simulink model "Tracking"  (Simulink 8.9)
settings: Solver=VariableStepAuto  StartTime=0.0  StopTime=1  RelTol=1e-3
undefined symbols (not defined in the file): magnitude
libraries: commfilt2 x24, simulink x20, dspmtrx3 x12, dspswit3 x8
(part 1 of 2)
settings Model: SuppressorTable="22 serialization::archive 11 0 6 0 0 16 64 0 0 0 0 6 0 0 1 0 79 Tracking Loop/Tracking Loops/Tracking Loop2/PRN Generator /Counter Free-Running 0 6 0 0 2 8 0 0 0 0 6 40 SimulinkFixedPoint:util:Overflowoccurred 0 0 0 6 0  0  0 0 0 0 8 20160523 0 0 0 10 57 55 0 1 41 Simulink:DataType:WarningOverFlowDetected 0 0 0  0  8 20160523 0 10 57 55 0 1 1 0 79 Tracking Loop/Tracking Loops/Tracking Loop4/PRN Generator /Counter Free-Running 2 8 0 40 SimulinkFixedPoint:util:Overflowoccurred 0 0 0  0  8 20160523 0 10 57 55 0 1 41 Simulink:DataType:WarningOverFlowDetected 0 0 0  0  8 20160523 0 10 57 55 0 1 1 0 84 Tracking/Tracking Loop/Tracking Loops/Tracking Loop1/Oscillator/Counter Free-Running 2 8 0 40 SimulinkFixedPoint:util:Overflowoccurred 0 0 0  0  8 20160523 0 10 57 55 0 1 41 Simulink:DataType:WarningOverFlowDetected 0 0 0  0  8 20160523 0 10 57 55 0 1 1 0 75 Tracking Loop/Tracking Loops/Tracking Loop1/Oscillator/Counter Free-Running 2 8 0 40 SimulinkFixedPoint:util:Overflowoccurred 0 0 0  0  8 20160523 0 10 57 55 0 1 41 Simulink:DataType:WarningOverFlowDetected 0 0 0  0  8 20160523 0 10 57 55 0 1 1 0 88 Tracking/Tracking Loop/Tracking Loops/Tracking Loop1/PRN Generator /Counter Free-Running 2 8 0 40 SimulinkFixedPoint:util:Overflowoccurred 0 0 0  0  8 20160523 0 10 57 55 0 1 41 Simulink:DataType:WarningOverFlowDetected 0 0 0  0  8 20160523 0 10 57 55 0 1 1 0 75 Tracking Loop/Tracking Loops/Tracking Loop4/Oscillator/Counter Free-Running 2 8 0 40 SimulinkFixedPoint:util:Overflowoccurred 0 0 0  0  8 20160523 0 10 57 55 0 1 41 Simulink:DataType:WarningOverFlowDetected 0 0 0  0  8 20160523 0 10 57 55 0 1 1 0 79 Tracking Loop/Tracking Loops/Tracking Loop3/PRN Generator /Counter Free-Running 2 8 0 40 SimulinkFixedPoint:util:Overflowoccurred 0 0 0  0  8 20160523 0 10 57 55 0 1 41 Simulink:DataType:WarningOverFlowDetected 0 0 0  0  8 20160523 0 10 57 55 0 1 1 0 75 Tracking Loop/Tracking Loops/Tracking Loop3/Oscillator/Counter Free-Running 2 8 0 40 SimulinkFixedPoint:util:Overflowoccurred 0 0 0  0  8 20160523 0 10 57 55 0 1 41 Simulink:DataType:WarningOverFlowDetected 0 0 0  0  8 20160523 0 10 57 55 0 1 1 0 75 Tracking Loop/Tracking Loops/Tracking Loop2/Oscillator/Counter Free-Running 2 8 0 40 SimulinkFixedPoint:util:Overflowoccurred 0 0 0  0  8 20160523 0 10 57 55 0 1 41 Simulink:DataType:WarningOverFlowDetected 0 0 0  0  8 20160523 0 10 57 55 0 1 1 0 79 Tracking Loop/Tracking Loops/Tracking Loop1/PRN Generator /Counter Free-Running 2 8 0 40 SimulinkFixedPoint:util:Overflowoccurred 0 0 0  0  8 20160523 0 10 57 55 0 1 41 Simulink:DataType:WarningOverFlowDetected 0 0 0  0  8 20160523 0 10 57 55 0 1 1 0 84 Tracking/Tracking Loop/Tracking Loops/Tracking Loop2/Oscillator/Counter Free-Running 2 8 0 40 SimulinkFixedPoint:util:Overflowoccurred 0 0 0  0  8 20160523 0 10 57 55 0 1 41 Simulink:DataType:WarningOverFlowDetected 0 0 0  0  8 20160523 0 10 57 55 0 1 1 0 88 Tracking/Tracking Loop/Tracking Loops/Tracking Loop2/PRN Generator /Counter Free-Running 2 8 0 40 SimulinkFixedPoint:util:Overflowoccurred 0 0 0  0  8 20160523 0 10 57 55 0 1 41 Simulink:DataType:WarningOverFlowDetected 0 0 0  0  8 20160523 0 10 57 55 0 1 1 0 84 Tracking/Tracking Loop/Tracking Loops/Tracking Loop3/Oscillator/Counter Free-Running 2 8 0 40 SimulinkFixedPoint:util:Overflowoccurred 0 0 0  0  8 20160523 0 10 57 55 0 1 41 Simulink:DataType:WarningOverFlowDetected 0 0 0  0  8 20160523 0 10 57 55 0 1 1 0 88 Tracking/Tracking Loop/Tracking Loops/Tracking Loop3/PRN Generator /Counter Free-Running 2 8 0 40 SimulinkFixedPoint:util:Overflowoccurred 0 0 0  0  8 20160523 0 10 57 55 0 1 41 Simulink:DataType:WarningOverFlowDetected 0 0 0  0  8 20160523 0 10 57 55 0 1 1 0 84 Tracking/Tracking Loop/Tracking Loops/Tracking Loop4/Oscillator/Counter Free-Running 2 8 0 40 SimulinkFixedPoint:util:Overflowoccurred 0 0 0  0  8 20160523 0 10 57 55 0 1 41 Simulink:DataType:WarningOverFlowDetected 0 0 0  0  8 20160523 0 10 57 55 0 1 1 0 88 Tracking/Tracking Loop/Tracking Loops/Tracking Loop4/PRN Generator /Counter Free-Running 2 8 0 40 SimulinkFixedPoint:util:Overflowoccurred 0 0 0  0  8 20160523 0 10 57 55 0 1 41 Simulink:DataType:WarningOverFlowDetected 0 0 0  0  8 20160523 0 10 57 55 0 1"  Creator=Alam  LastModifiedBy=Alam
settings DataIOCC: LimitDataPoints=off  SaveFormat=Dataset  SignalLoggingSaveFormat=Dataset
settings OptimizationCC: LifeSpan=auto
settings DebuggingCC: UnderspecifiedInitializationDetection=Simplified  MergeDetectMultiDrivingBlocksExec=error  FcnCallInpInsideContextMsg=error  StateNameClashWarn=none  SFUnexpectedBacktrackingDiag=error  SFNoUnconditionalDefaultTransitionDiag=error  SFExecutionAtInitializationDiag=warning
settings HardwareCC: ProdBitPerPointer=64  ProdBitPerSizeT=64  ProdBitPerPtrDiffT=64  ProdLargestAtomicFloat=Float  ProdIntDivRoundTo=Zero  ProdEndianess=LittleEndian  ProdWordSize=64  ProdHWDeviceType=Intel->x86-64 (Windows64)
settings ModelReferenceCC: PropagateSignalLabelsOutOfModel=on
settings GRTTargetCC: TargetLangStandard=C99 (ISO)  GeneratePreprocessorConditionals=Use local settings  CombineOutputUpdateFcns=on  GRTInterface=off
settings ConfigComp: CovMetricSettings=dwe  CovHtmlReporting=off  CovSaveCumulativeToWorkspaceVar=off  CovSaveSingleToWorkspaceVar=off  CovExternalEMLEnable=on

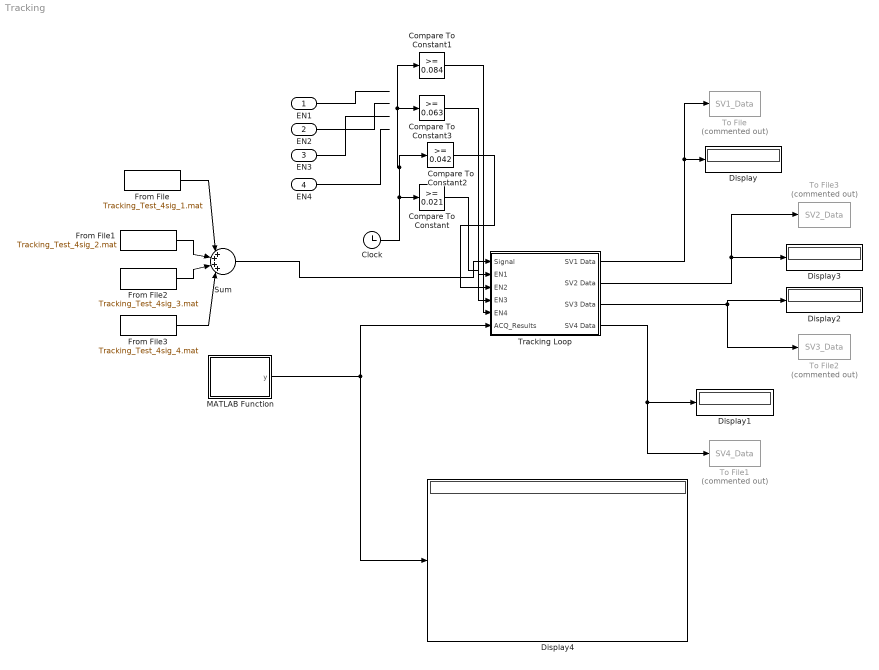
== system Tracking ==
  EN1 : Inport
  EN2 : Inport  Port=2
  EN3 : Inport  Port=3
  EN4 : Inport  Port=4
  Clock : Clock
  Compare To Constant : simulink/Logic and Bit Operations/Compare To Constant  relop=>=  const=0.021  OutDataTypeStr=boolean
  Compare To Constant1 : simulink/Logic and Bit Operations/Compare To Constant  relop=>=  const=0.084  OutDataTypeStr=boolean
  Compare To Constant2 : simulink/Logic and Bit Operations/Compare To Constant  relop=>=  const=0.042  OutDataTypeStr=boolean
  Compare To Constant3 : simulink/Logic and Bit Operations/Compare To Constant  relop=>=  const=0.063  OutDataTypeStr=boolean
  Display{,1..4} (5 alike) : Display
  From File : FromFile  FileName=Tracking_Test_4sig_1.mat  SampleTime=0
  From File1 : FromFile  FileName=Tracking_Test_4sig_2.mat  SampleTime=0
  From File2 : FromFile  FileName=Tracking_Test_4sig_3.mat  SampleTime=0
  From File3 : FromFile  FileName=Tracking_Test_4sig_4.mat  SampleTime=0
  MATLAB Function : MATLAB Function
  Sum : Sum  Inputs=|++++|
  To File : ToFile  Commented=on  Filename=SV1_Data  MatrixName=SV1  SampleTime=0.01
  To File1 : ToFile  Commented=on  Filename=SV4_Data  MatrixName=SV4  SampleTime=0.01
  To File2 : ToFile  Commented=on  Filename=SV3_Data  MatrixName=SV3  SampleTime=0.01
  To File3 : ToFile  Commented=on  Filename=SV2_Data  MatrixName=SV2  SampleTime=0.01
  Tracking Loop : Subsystem  TreatAsAtomicUnit=on
  wires:
  Tracking Loop/3(SV3 Data) -> Display2/1, To File2/1
  Tracking Loop/4(SV4 Data) -> To File1/1, Display1/1
  Tracking Loop/2(SV2 Data) -> Display3/1, To File3/1
  Tracking Loop/1(SV1 Data) -> Display/1, To File/1
  Compare To Constant2/1 -> Tracking Loop/3(EN2)
  Compare To Constant/1 -> Tracking Loop/2(EN1)
  Clock/1 -> Compare To Constant1/1, Compare To Constant3/1, Compare To Constant2/1, Compare To Constant/1
  Compare To Constant3/1 -> Tracking Loop/4(EN3)
  Compare To Constant1/1 -> Tracking Loop/5(EN4)
  Sum/1 -> Tracking Loop/1(Signal)
  From File2/1 -> Sum/3
  From File/1 -> Sum/1
  From File1/1 -> Sum/2
  From File3/1 -> Sum/4
  EN3/1 -> ?
  EN4/1 -> ?
  EN2/1 -> ?
  EN1/1 -> ?
  MATLAB Function/1(y) -> Tracking Loop/6(ACQ_Results), Display4/1

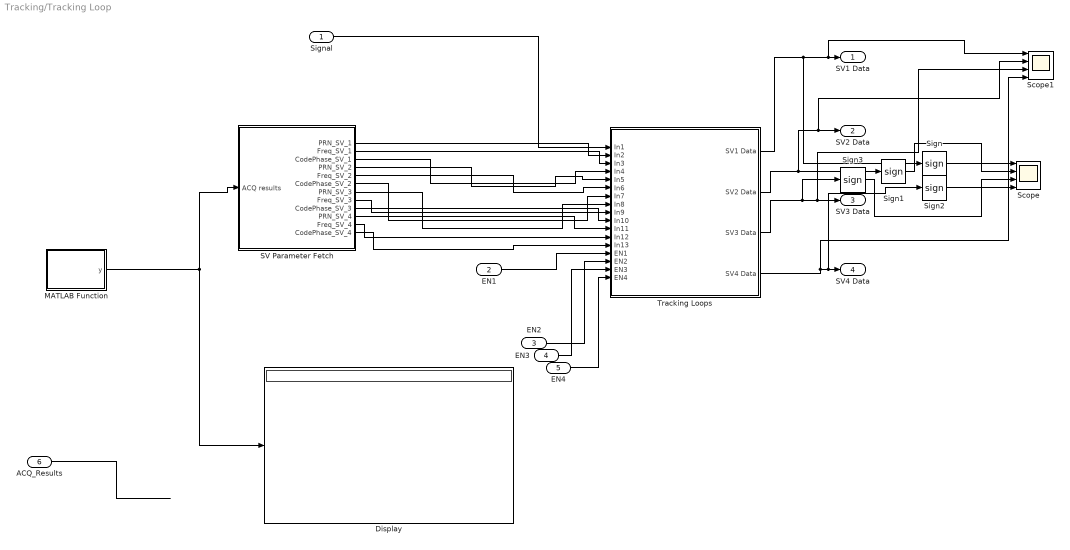
== system Tracking/Tracking Loop ==
  Signal : Inport
  EN1 : Inport  Port=2
  EN2 : Inport  Port=3
  EN3 : Inport  Port=4
  EN4 : Inport  Port=5
  ACQ_Results : Inport  Port=6
  Display : Display
  MATLAB Function : MATLAB Function  TreatAsAtomicUnit=on
  SV Parameter Fetch : Subsystem
  Scope : Scope  NumInputPorts=4
  Scope1 : Scope  NumInputPorts=4
  Sign{,1..3} (4 alike) : Signum
  Tracking Loops : Subsystem
  SV1 Data : Outport
  SV2 Data : Outport  Port=2
  SV3 Data : Outport  Port=3
  SV4 Data : Outport  Port=4
  wires:
  Signal/1 -> Tracking Loops/1(In1)
  Tracking Loops/1(SV1 Data) -> Sign/1, Scope1/1, SV1 Data/1
  Tracking Loops/2(SV2 Data) -> Scope1/2, SV2 Data/1, Sign1/1
  Tracking Loops/3(SV3 Data) -> Sign3/1, Scope1/3, SV3 Data/1
  Tracking Loops/4(SV4 Data) -> Scope1/4, Sign2/1, SV4 Data/1
  Sign/1 -> Scope/1
  Sign1/1 -> Scope/2
  Sign2/1 -> Scope/4
  Sign3/1 -> Scope/3
  SV Parameter Fetch/12(CodePhase_SV_4) -> Tracking Loops/13(In13)
  SV Parameter Fetch/11(Freq_SV_4) -> Tracking Loops/12(In12)
  SV Parameter Fetch/10(PRN_SV_4) -> Tracking Loops/11(In11)
  SV Parameter Fetch/9(CodePhase_SV_3) -> Tracking Loops/10(In10)
  SV Parameter Fetch/8(Freq_SV_3) -> Tracking Loops/9(In9)
  SV Parameter Fetch/7(PRN_SV_3) -> Tracking Loops/8(In8)
  SV Parameter Fetch/6(CodePhase_SV_2) -> Tracking Loops/7(In7)
  SV Parameter Fetch/5(Freq_SV_2) -> Tracking Loops/6(In6)
  SV Parameter Fetch/4(PRN_SV_2) -> Tracking Loops/5(In5)
  SV Parameter Fetch/3(CodePhase_SV_1) -> Tracking Loops/4(In4)
  SV Parameter Fetch/2(Freq_SV_1) -> Tracking Loops/3(In3)
  SV Parameter Fetch/1(PRN_SV_1) -> Tracking Loops/2(In2)
  MATLAB Function/1(y) -> SV Parameter Fetch/1(ACQ results), Display/1
  EN1/1 -> Tracking Loops/14(EN1)
  EN2/1 -> Tracking Loops/15(EN2)
  EN3/1 -> Tracking Loops/16(EN3)
  EN4/1 -> Tracking Loops/17(EN4)
  ACQ_Results/1 -> ?

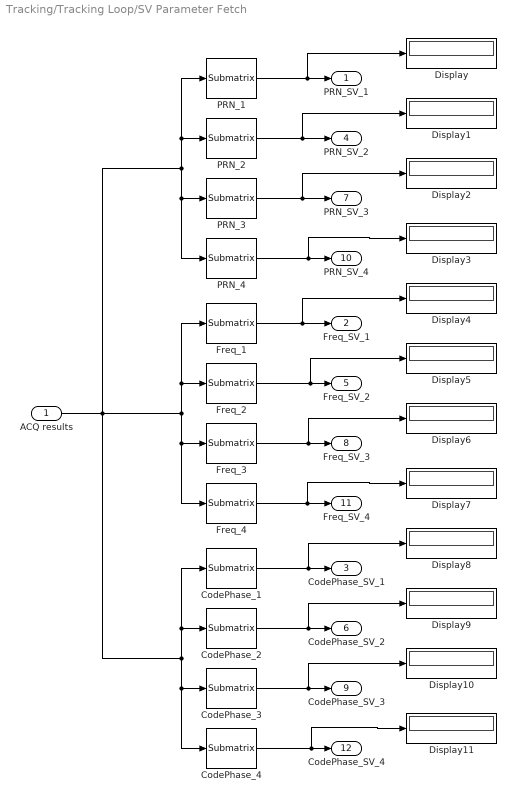
== system Tracking/Tracking Loop/SV Parameter Fetch ==
  ACQ results : Inport
  CodePhase_1 : dspmtrx3/Submatrix  RowSpan=One row  RowStartMode=Index  RowStartIndex=1  RowEndMode=Last  RowEndIndex=1  ColSpan=One column  ColStartMode=Index  ColStartIndex=4  ColEndMode=Last  ColEndIndex=1
  CodePhase_2 : dspmtrx3/Submatrix  RowSpan=One row  RowStartMode=Index  RowStartIndex=2  RowEndMode=Last  RowEndIndex=1  ColSpan=One column  ColStartMode=Index  ColStartIndex=4  ColEndMode=Last  ColEndIndex=1
  CodePhase_3 : dspmtrx3/Submatrix  RowSpan=One row  RowStartMode=Index  RowStartIndex=3  RowEndMode=Last  RowEndIndex=1  ColSpan=One column  ColStartMode=Index  ColStartIndex=4  ColEndMode=Last  ColEndIndex=1
  CodePhase_4 : dspmtrx3/Submatrix  RowSpan=One row  RowStartMode=Index  RowStartIndex=4  RowEndMode=Last  RowEndIndex=1  ColSpan=One column  ColStartMode=Index  ColStartIndex=4  ColEndMode=Last  ColEndIndex=1
  Display{,1..11} (12 alike) : Display
  Freq_1 : dspmtrx3/Submatrix  RowSpan=One row  RowStartMode=Index  RowStartIndex=1  RowEndMode=Last  RowEndIndex=1  ColSpan=One column  ColStartMode=Index  ColStartIndex=3  ColEndMode=Last  ColEndIndex=1
  Freq_2 : dspmtrx3/Submatrix  RowSpan=One row  RowStartMode=Index  RowStartIndex=2  RowEndMode=Last  RowEndIndex=1  ColSpan=One column  ColStartMode=Index  ColStartIndex=3  ColEndMode=Last  ColEndIndex=1
  Freq_3 : dspmtrx3/Submatrix  RowSpan=One row  RowStartMode=Index  RowStartIndex=3  RowEndMode=Last  RowEndIndex=1  ColSpan=One column  ColStartMode=Index  ColStartIndex=3  ColEndMode=Last  ColEndIndex=1
  Freq_4 : dspmtrx3/Submatrix  RowSpan=One row  RowStartMode=Index  RowStartIndex=4  RowEndMode=Last  RowEndIndex=1  ColSpan=One column  ColStartMode=Index  ColStartIndex=3  ColEndMode=Last  ColEndIndex=1
  PRN_1 : dspmtrx3/Submatrix  RowSpan=One row  RowStartMode=Index  RowStartIndex=1  RowEndMode=Last  RowEndIndex=1  ColSpan=One column  ColStartMode=Index  ColStartIndex=2  ColEndMode=Last  ColEndIndex=1
  PRN_2 : dspmtrx3/Submatrix  RowSpan=One row  RowStartMode=Index  RowStartIndex=2  RowEndMode=Last  RowEndIndex=1  ColSpan=One column  ColStartMode=Index  ColStartIndex=2  ColEndMode=Last  ColEndIndex=1
  PRN_3 : dspmtrx3/Submatrix  RowSpan=One row  RowStartMode=Index  RowStartIndex=3  RowEndMode=Last  RowEndIndex=1  ColSpan=One column  ColStartMode=Index  ColStartIndex=2  ColEndMode=Last  ColEndIndex=1
  PRN_4 : dspmtrx3/Submatrix  RowSpan=One row  RowStartMode=Index  RowStartIndex=4  RowEndMode=Last  RowEndIndex=1  ColSpan=One column  ColStartMode=Index  ColStartIndex=2  ColEndMode=Last  ColEndIndex=1
  PRN_SV_1 : Outport
  Freq_SV_1 : Outport  Port=2
  CodePhase_SV_1 : Outport  Port=3
  PRN_SV_2 : Outport  Port=4
  Freq_SV_2 : Outport  Port=5
  CodePhase_SV_2 : Outport  Port=6
  PRN_SV_3 : Outport  Port=7
  Freq_SV_3 : Outport  Port=8
  CodePhase_SV_3 : Outport  Port=9
  PRN_SV_4 : Outport  Port=10
  Freq_SV_4 : Outport  Port=11
  CodePhase_SV_4 : Outport  Port=12
  wires:
  ACQ results/1 -> CodePhase_4/1, CodePhase_3/1, CodePhase_2/1, CodePhase_1/1, Freq_4/1, Freq_3/1, Freq_2/1, Freq_1/1, PRN_4/1, PRN_3/1, PRN_2/1, PRN_1/1
  PRN_1/1 -> Display/1, PRN_SV_1/1
  PRN_2/1 -> Display1/1, PRN_SV_2/1
  PRN_3/1 -> Display2/1, PRN_SV_3/1
  PRN_4/1 -> Display3/1, PRN_SV_4/1
  Freq_1/1 -> Display4/1, Freq_SV_1/1
  Freq_2/1 -> Display5/1, Freq_SV_2/1
  Freq_3/1 -> Display6/1, Freq_SV_3/1
  Freq_4/1 -> Display7/1, Freq_SV_4/1
  CodePhase_1/1 -> Display8/1, CodePhase_SV_1/1
  CodePhase_2/1 -> Display9/1, CodePhase_SV_2/1
  CodePhase_3/1 -> Display10/1, CodePhase_SV_3/1
  CodePhase_4/1 -> Display11/1, CodePhase_SV_4/1

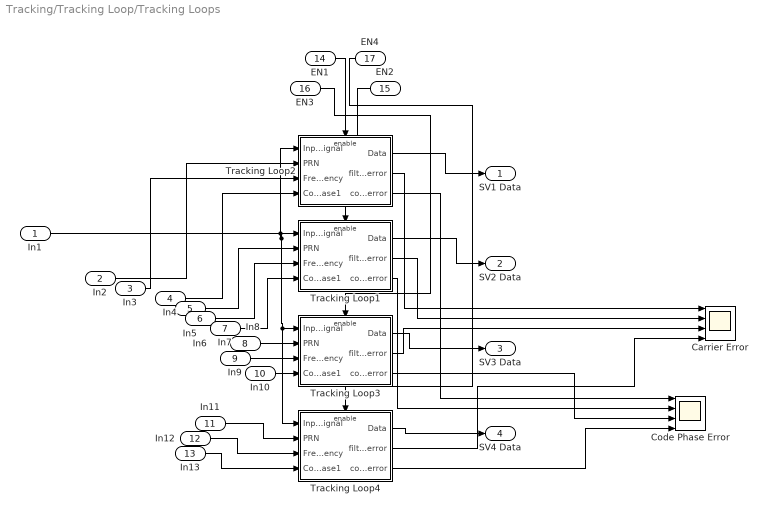
== system Tracking/Tracking Loop/Tracking Loops ==
  In1 : Inport
  In2 : Inport  Port=2
  In3 : Inport  Port=3
  In4 : Inport  Port=4
  In5 : Inport  Port=5
  In6 : Inport  Port=6
  In7 : Inport  Port=7
  In8 : Inport  Port=8
  In9 : Inport  Port=9
  In10 : Inport  Port=10
  In11 : Inport  Port=11
  In12 : Inport  Port=12
  In13 : Inport  Port=13
  EN1 : Inport  Port=14
  EN2 : Inport  Port=15
  EN3 : Inport  Port=16
  EN4 : Inport  Port=17
  Carrier Error : Scope  NumInputPorts=4
  Code Phase Error : Scope  NumInputPorts=4
  Tracking Loop1 : Subsystem  TreatAsAtomicUnit=on
      settings: PropExecContextOutsideSubsystem=on
  Tracking Loop2 : Subsystem  TreatAsAtomicUnit=on
  Tracking Loop3 : Subsystem  TreatAsAtomicUnit=on
      settings: PropExecContextOutsideSubsystem=on
  Tracking Loop4 : Subsystem  TreatAsAtomicUnit=on
      settings: PropExecContextOutsideSubsystem=on
  SV1 Data : Outport
  SV2 Data : Outport  Port=2
  SV3 Data : Outport  Port=3
  SV4 Data : Outport  Port=4
  wires:
  In1/1 -> Tracking Loop2/1(Input Signal), Tracking Loop1/1(Input Signal), Tracking Loop4/1(Input Signal), Tracking Loop3/1(Input Signal)
  Tracking Loop2/1(Data) -> SV1 Data/1
  Tracking Loop4/1(Data) -> SV4 Data/1
  Tracking Loop3/1(Data) -> SV3 Data/1
  In12/1 -> Tracking Loop4/3(Frequency)
  In3/1 -> Tracking Loop2/3(Frequency)
  In4/1 -> Tracking Loop2/4(Code Phase1)
  In6/1 -> Tracking Loop1/3(Frequency)
  In13/1 -> Tracking Loop4/4(Code Phase1)
  In9/1 -> Tracking Loop3/3(Frequency)
  In8/1 -> Tracking Loop3/2(PRN)
  In11/1 -> Tracking Loop4/2(PRN)
  In5/1 -> Tracking Loop1/2(PRN)
  In10/1 -> Tracking Loop3/4(Code Phase1)
  In2/1 -> Tracking Loop2/2(PRN)
  In7/1 -> Tracking Loop1/4(Code Phase1)
  Tracking Loop1/1(Data) -> SV2 Data/1
  Tracking Loop2/2(filter error) -> Carrier Error/1
  Tracking Loop1/2(filter error) -> Carrier Error/2
  Tracking Loop3/2(filter error) -> Carrier Error/3
  Tracking Loop4/2(filter error) -> Carrier Error/4
  Tracking Loop3/3(code_phase_error) -> Code Phase Error/3
  Tracking Loop4/3(code_phase_error) -> Code Phase Error/4
  Tracking Loop2/3(code_phase_error) -> Code Phase Error/1
  Tracking Loop1/3(code_phase_error) -> Code Phase Error/2
  EN1/1 -> Tracking Loop2/Enable
  EN2/1 -> Tracking Loop1/Enable
  EN3/1 -> Tracking Loop3/Enable
  EN4/1 -> Tracking Loop4/Enable

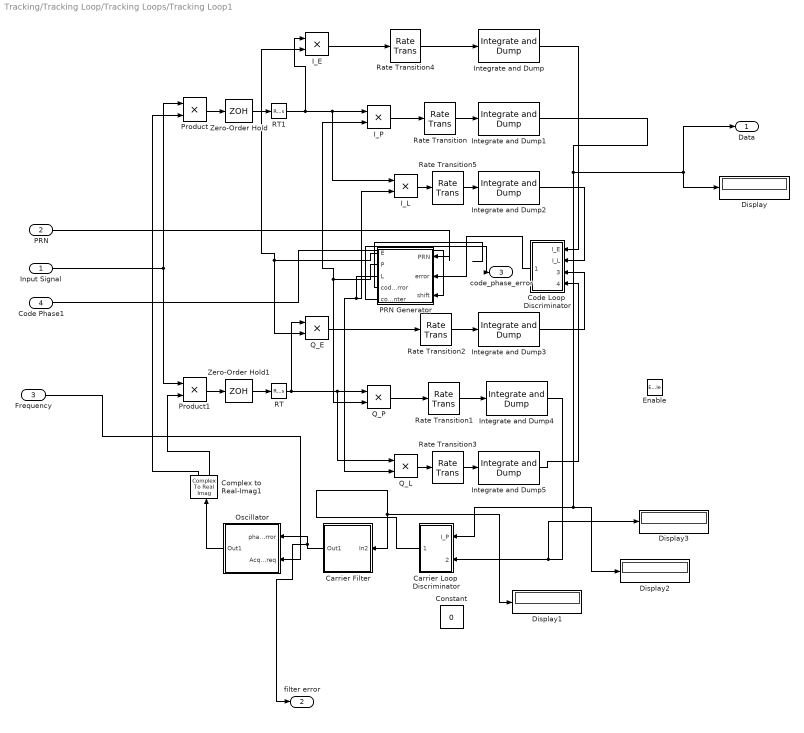
== system Tracking/Tracking Loop/Tracking Loops/Tracking Loop1 ==
  Input Signal : Inport
  PRN : Inport  Port=2
  Frequency : Inport  Port=3
  Code Phase1 : Inport  Port=4
  Enable : EnablePort
  Carrier Filter : Subsystem
  "Carrier Loop  Discriminator " : Subsystem
  Code Loop  Discriminator : Subsystem
  Complex to Real-Imag1 : ComplexToRealImag
  Constant : Constant  Value=0  SampleTime=0.001
  Display{,1..3} (4 alike) : Display
  I_E : Product
  I_L : Product
  "I_P " : Product
  Integrate and Dump{,1..5} (6 alike) : commfilt2/Integrate and Dump  obssamples=32768  offsetsamples=0  nodump=off  roundingMode=Floor  overflowMode=off  outputDataTypeStr=Inherit: Same as accumulator  outputLastDataTypeStr=Inherit: Same as accumulator
      settings: SourceProductName=Communications System Toolbox
  Oscillator : Subsystem
  "PRN Generator " : Subsystem
  Product : Product
  Product1 : Product
  Q_E : Product
  Q_L : Product
  Q_P : Product
  RT : RateTransition
  RT1 : RateTransition
  Rate Transition{,1..5} (6 alike) : RateTransition  OutPortSampleTime=3.0517578125e-8
  Zero-Order Hold : ZeroOrderHold  SampleTime=3.0517578125e-8
  Zero-Order Hold1 : ZeroOrderHold  SampleTime=3.0517578125e-8
  Data : Outport
  filter error : Outport  Port=2
  code_phase_error : Outport  Port=3
  wires:
  I_L/1 -> Rate Transition5/1
  "PRN Generator "/3(L) -> Q_L/2, I_L/2
  Q_E/1 -> Rate Transition2/1
  Q_L/1 -> Rate Transition3/1
  "PRN Generator "/2(P) -> "I_P "/2, Q_P/2
  Q_P/1 -> Rate Transition1/1
  "I_P "/1 -> Rate Transition/1
  "Carrier Loop  Discriminator "/1(theta) -> Carrier Filter/1(In2), Display1/1
  Rate Transition/1 -> Integrate and Dump1/1
  Rate Transition4/1 -> Integrate and Dump/1
  RT/1 -> Q_L/1, Q_P/1, Q_E/1
  Code Phase1/1 -> "PRN Generator "/3(shift)
  Product/1 -> Zero-Order Hold/1
  PRN/1 -> "PRN Generator "/1(PRN)
  Complex to Real-Imag1/2 -> Product1/2
  Input Signal/1 -> Product1/1, Product/1
  Complex to Real-Imag1/1 -> Product/2
  I_E/1 -> Rate Transition4/1
  Integrate and Dump/1 -> Code Loop  Discriminator/1(I_E)
  Integrate and Dump5/1 -> Code Loop  Discriminator/4(Q_L)
  Integrate and Dump3/1 -> Code Loop  Discriminator/3(Q_E)
  "PRN Generator "/1(E) -> I_E/2, Q_E/2
  Integrate and Dump2/1 -> Code Loop  Discriminator/2(I_L)
  Rate Transition1/1 -> Integrate and Dump4/1
  Rate Transition3/1 -> Integrate and Dump5/1
  Rate Transition2/1 -> Integrate and Dump3/1
  Rate Transition5/1 -> Integrate and Dump2/1
  Frequency/1 -> Oscillator/2(Acq Freq)
  Product1/1 -> Zero-Order Hold1/1
  Zero-Order Hold/1 -> RT1/1
  RT1/1 -> I_E/1, I_L/1, "I_P "/1
  Zero-Order Hold1/1 -> RT/1
  Oscillator/1(Out1) -> Complex to Real-Imag1/1
  Carrier Filter/1(Out1) -> filter error/1, Oscillator/1(phase error)
  Integrate and Dump4/1 -> "Carrier Loop  Discriminator "/2(Q_P), Display3/1
  Integrate and Dump1/1 -> Display/1, Data/1, "Carrier Loop  Discriminator "/1(I_P), Display2/1
  "PRN Generator "/4(code_phase_error) -> ?
  "PRN Generator "/5(code_phase_counter) -> code_phase_error/1
  Code Loop  Discriminator/1(error) -> "PRN Generator "/2(error)

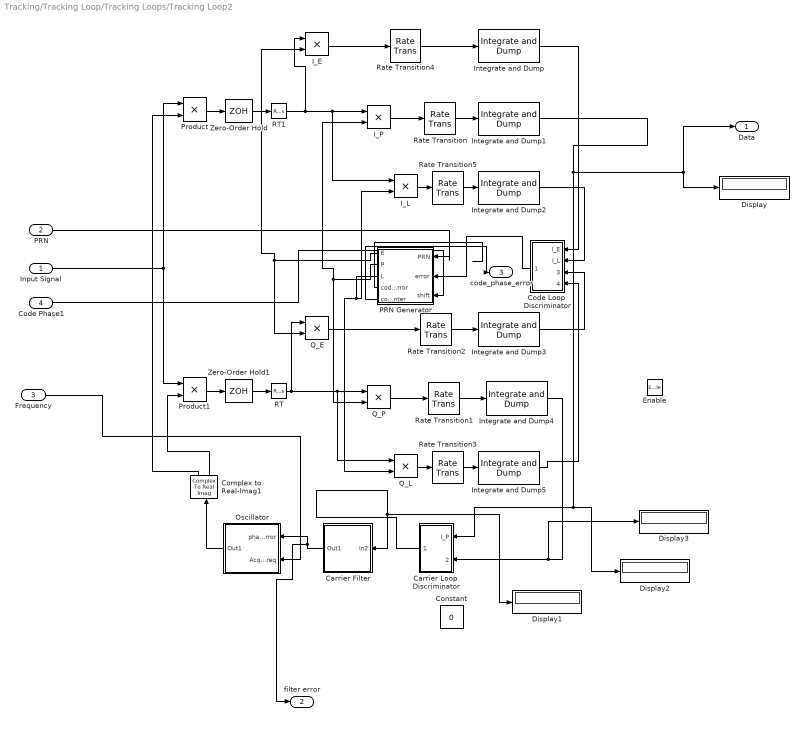
== system Tracking/Tracking Loop/Tracking Loops/Tracking Loop2 ==
  Input Signal : Inport
  PRN : Inport  Port=2
  Frequency : Inport  Port=3
  Code Phase1 : Inport  Port=4
  Enable : EnablePort
  Carrier Filter : Subsystem
      settings: MinAlgLoopOccurrences=on
  "Carrier Loop  Discriminator " : Subsystem
  Code Loop  Discriminator : Subsystem
      settings: MinAlgLoopOccurrences=on
  Complex to Real-Imag1 : ComplexToRealImag
  Constant : Constant  Value=0  SampleTime=0.001
  Display{,1..3} (4 alike) : Display
  I_E : Product
  I_L : Product
  "I_P " : Product
  Integrate and Dump{,1..5} (6 alike) : commfilt2/Integrate and Dump  obssamples=32768  offsetsamples=0  nodump=off  roundingMode=Floor  overflowMode=off  outputDataTypeStr=Inherit: Same as accumulator  outputLastDataTypeStr=Inherit: Same as accumulator
      settings: SourceProductName=Communications System Toolbox
  Oscillator : Subsystem
  "PRN Generator " : Subsystem
      settings: MinAlgLoopOccurrences=on
  Product : Product
  Product1 : Product
  Q_E : Product
  Q_L : Product
  Q_P : Product
  RT : RateTransition
  RT1 : RateTransition
  Rate Transition{,1..5} (6 alike) : RateTransition  OutPortSampleTime=3.0517578125e-8
  Zero-Order Hold : ZeroOrderHold  SampleTime=3.0517578125e-8
  Zero-Order Hold1 : ZeroOrderHold  SampleTime=3.0517578125e-8
  Data : Outport
  filter error : Outport  Port=2
  code_phase_error : Outport  Port=3
  wires:
  I_L/1 -> Rate Transition5/1
  "PRN Generator "/3(L) -> Q_L/2, I_L/2
  Q_E/1 -> Rate Transition2/1
  Q_L/1 -> Rate Transition3/1
  "PRN Generator "/2(P) -> "I_P "/2, Q_P/2
  Q_P/1 -> Rate Transition1/1
  "I_P "/1 -> Rate Transition/1
  "Carrier Loop  Discriminator "/1(theta) -> Carrier Filter/1(In2), Display1/1
  Rate Transition/1 -> Integrate and Dump1/1
  Rate Transition4/1 -> Integrate and Dump/1
  RT/1 -> Q_L/1, Q_P/1, Q_E/1
  Code Phase1/1 -> "PRN Generator "/3(shift)
  Product/1 -> Zero-Order Hold/1
  PRN/1 -> "PRN Generator "/1(PRN)
  Complex to Real-Imag1/2 -> Product1/2
  Input Signal/1 -> Product1/1, Product/1
  Complex to Real-Imag1/1 -> Product/2
  I_E/1 -> Rate Transition4/1
  Integrate and Dump/1 -> Code Loop  Discriminator/1(I_E)
  Integrate and Dump5/1 -> Code Loop  Discriminator/4(Q_L)
  Integrate and Dump3/1 -> Code Loop  Discriminator/3(Q_E)
  "PRN Generator "/1(E) -> I_E/2, Q_E/2
  Integrate and Dump2/1 -> Code Loop  Discriminator/2(I_L)
  Rate Transition1/1 -> Integrate and Dump4/1
  Rate Transition3/1 -> Integrate and Dump5/1
  Rate Transition2/1 -> Integrate and Dump3/1
  Rate Transition5/1 -> Integrate and Dump2/1
  Frequency/1 -> Oscillator/2(Acq Freq)
  Product1/1 -> Zero-Order Hold1/1
  Zero-Order Hold/1 -> RT1/1
  RT1/1 -> I_E/1, I_L/1, "I_P "/1
  Zero-Order Hold1/1 -> RT/1
  Oscillator/1(Out1) -> Complex to Real-Imag1/1
  Carrier Filter/1(Out1) -> filter error/1, Oscillator/1(phase error)
  Integrate and Dump4/1 -> "Carrier Loop  Discriminator "/2(Q_P), Display3/1
  Integrate and Dump1/1 -> Display/1, Data/1, "Carrier Loop  Discriminator "/1(I_P), Display2/1
  "PRN Generator "/4(code_phase_error) -> ?
  "PRN Generator "/5(code_phase_counter) -> code_phase_error/1
  Code Loop  Discriminator/1(error) -> "PRN Generator "/2(error)

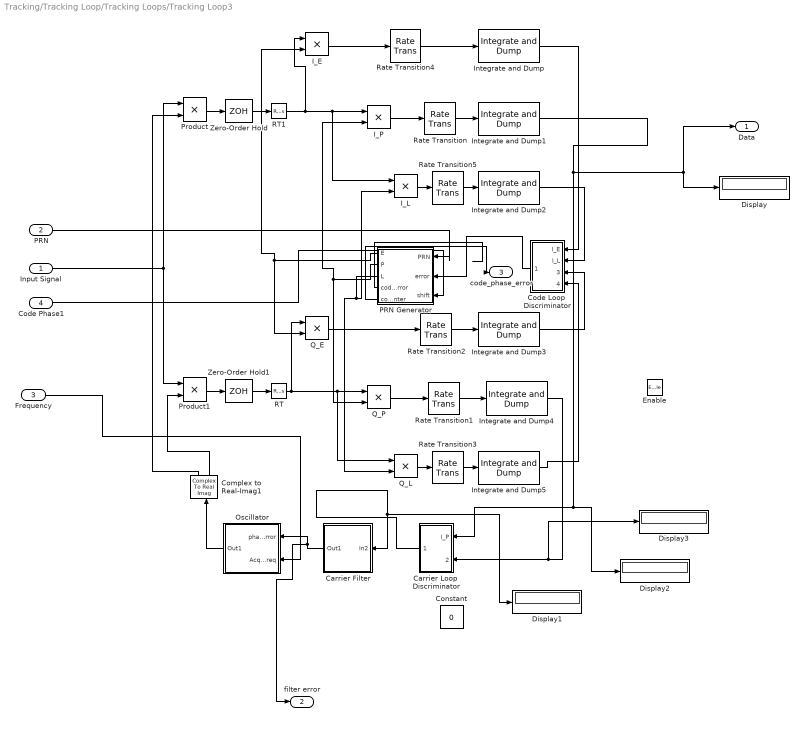
== system Tracking/Tracking Loop/Tracking Loops/Tracking Loop3 ==
  Input Signal : Inport
  PRN : Inport  Port=2
  Frequency : Inport  Port=3
  Code Phase1 : Inport  Port=4
  Enable : EnablePort
  Carrier Filter : Subsystem
  "Carrier Loop  Discriminator " : Subsystem
  Code Loop  Discriminator : Subsystem
  Complex to Real-Imag1 : ComplexToRealImag
  Constant : Constant  Value=0  SampleTime=0.001
  Display{,1..3} (4 alike) : Display
  I_E : Product
  I_L : Product
  "I_P " : Product
  Integrate and Dump{,1..5} (6 alike) : commfilt2/Integrate and Dump  obssamples=32768  offsetsamples=0  nodump=off  roundingMode=Floor  overflowMode=off  outputDataTypeStr=Inherit: Same as accumulator  outputLastDataTypeStr=Inherit: Same as accumulator
      settings: SourceProductName=Communications System Toolbox
  Oscillator : Subsystem
  "PRN Generator " : Subsystem
  Product : Product
  Product1 : Product
  Q_E : Product
  Q_L : Product
  Q_P : Product
  RT : RateTransition
  RT1 : RateTransition
  Rate Transition{,1..5} (6 alike) : RateTransition  OutPortSampleTime=3.0517578125e-8
  Zero-Order Hold : ZeroOrderHold  SampleTime=3.0517578125e-8
  Zero-Order Hold1 : ZeroOrderHold  SampleTime=3.0517578125e-8
  Data : Outport
  filter error : Outport  Port=2
  code_phase_error : Outport  Port=3
  wires:
  I_L/1 -> Rate Transition5/1
  "PRN Generator "/3(L) -> Q_L/2, I_L/2
  Q_E/1 -> Rate Transition2/1
  Q_L/1 -> Rate Transition3/1
  "PRN Generator "/2(P) -> "I_P "/2, Q_P/2
  Q_P/1 -> Rate Transition1/1
  "I_P "/1 -> Rate Transition/1
  "Carrier Loop  Discriminator "/1(theta) -> Carrier Filter/1(In2), Display1/1
  Rate Transition/1 -> Integrate and Dump1/1
  Rate Transition4/1 -> Integrate and Dump/1
  RT/1 -> Q_L/1, Q_P/1, Q_E/1
  Code Phase1/1 -> "PRN Generator "/3(shift)
  Product/1 -> Zero-Order Hold/1
  PRN/1 -> "PRN Generator "/1(PRN)
  Complex to Real-Imag1/2 -> Product1/2
  Input Signal/1 -> Product1/1, Product/1
  Complex to Real-Imag1/1 -> Product/2
  I_E/1 -> Rate Transition4/1
  Integrate and Dump/1 -> Code Loop  Discriminator/1(I_E)
  Integrate and Dump5/1 -> Code Loop  Discriminator/4(Q_L)
  Integrate and Dump3/1 -> Code Loop  Discriminator/3(Q_E)
  "PRN Generator "/1(E) -> I_E/2, Q_E/2
  Integrate and Dump2/1 -> Code Loop  Discriminator/2(I_L)
  Rate Transition1/1 -> Integrate and Dump4/1
  Rate Transition3/1 -> Integrate and Dump5/1
  Rate Transition2/1 -> Integrate and Dump3/1
  Rate Transition5/1 -> Integrate and Dump2/1
  Frequency/1 -> Oscillator/2(Acq Freq)
  Product1/1 -> Zero-Order Hold1/1
  Zero-Order Hold/1 -> RT1/1
  RT1/1 -> I_E/1, I_L/1, "I_P "/1
  Zero-Order Hold1/1 -> RT/1
  Oscillator/1(Out1) -> Complex to Real-Imag1/1
  Carrier Filter/1(Out1) -> filter error/1, Oscillator/1(phase error)
  Integrate and Dump4/1 -> "Carrier Loop  Discriminator "/2(Q_P), Display3/1
  Integrate and Dump1/1 -> Display/1, Data/1, "Carrier Loop  Discriminator "/1(I_P), Display2/1
  "PRN Generator "/4(code_phase_error) -> ?
  "PRN Generator "/5(code_phase_counter) -> code_phase_error/1
  Code Loop  Discriminator/1(error) -> "PRN Generator "/2(error)

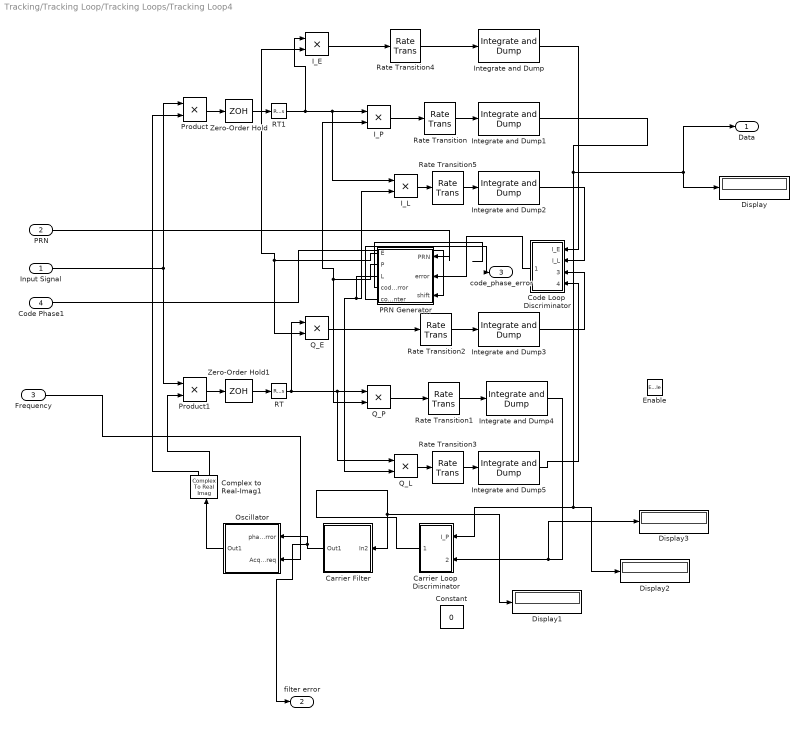
== system Tracking/Tracking Loop/Tracking Loops/Tracking Loop4 ==
  Input Signal : Inport
  PRN : Inport  Port=2
  Frequency : Inport  Port=3
  Code Phase1 : Inport  Port=4
  Enable : EnablePort
  Carrier Filter : Subsystem
  "Carrier Loop  Discriminator " : Subsystem
  Code Loop  Discriminator : Subsystem
  Complex to Real-Imag1 : ComplexToRealImag
  Constant : Constant  Value=0  SampleTime=0.001
  Display{,1..3} (4 alike) : Display
  I_E : Product
  I_L : Product
  "I_P " : Product
  Integrate and Dump{,1..5} (6 alike) : commfilt2/Integrate and Dump  obssamples=32768  offsetsamples=0  nodump=off  roundingMode=Floor  overflowMode=off  outputDataTypeStr=Inherit: Same as accumulator  outputLastDataTypeStr=Inherit: Same as accumulator
      settings: SourceProductName=Communications System Toolbox
  Oscillator : Subsystem
  "PRN Generator " : Subsystem
  Product : Product
  Product1 : Product
  Q_E : Product
  Q_L : Product
  Q_P : Product
  RT : RateTransition
  RT1 : RateTransition
  Rate Transition{,1..5} (6 alike) : RateTransition  OutPortSampleTime=3.0517578125e-8
  Zero-Order Hold : ZeroOrderHold  SampleTime=3.0517578125e-8
  Zero-Order Hold1 : ZeroOrderHold  SampleTime=3.0517578125e-8
  Data : Outport
  filter error : Outport  Port=2
  code_phase_error : Outport  Port=3
  wires:
  I_L/1 -> Rate Transition5/1
  "PRN Generator "/3(L) -> Q_L/2, I_L/2
  Q_E/1 -> Rate Transition2/1
  Q_L/1 -> Rate Transition3/1
  "PRN Generator "/2(P) -> "I_P "/2, Q_P/2
  Q_P/1 -> Rate Transition1/1
  "I_P "/1 -> Rate Transition/1
  "Carrier Loop  Discriminator "/1(theta) -> Carrier Filter/1(In2), Display1/1
  Rate Transition/1 -> Integrate and Dump1/1
  Rate Transition4/1 -> Integrate and Dump/1
  RT/1 -> Q_L/1, Q_P/1, Q_E/1
  Code Phase1/1 -> "PRN Generator "/3(shift)
  Product/1 -> Zero-Order Hold/1
  PRN/1 -> "PRN Generator "/1(PRN)
  Complex to Real-Imag1/2 -> Product1/2
  Input Signal/1 -> Product1/1, Product/1
  Complex to Real-Imag1/1 -> Product/2
  I_E/1 -> Rate Transition4/1
  Integrate and Dump/1 -> Code Loop  Discriminator/1(I_E)
  Integrate and Dump5/1 -> Code Loop  Discriminator/4(Q_L)
  Integrate and Dump3/1 -> Code Loop  Discriminator/3(Q_E)
  "PRN Generator "/1(E) -> I_E/2, Q_E/2
  Integrate and Dump2/1 -> Code Loop  Discriminator/2(I_L)
  Rate Transition1/1 -> Integrate and Dump4/1
  Rate Transition3/1 -> Integrate and Dump5/1
  Rate Transition2/1 -> Integrate and Dump3/1
  Rate Transition5/1 -> Integrate and Dump2/1
  Frequency/1 -> Oscillator/2(Acq Freq)
  Product1/1 -> Zero-Order Hold1/1
  Zero-Order Hold/1 -> RT1/1
  RT1/1 -> I_E/1, I_L/1, "I_P "/1
  Zero-Order Hold1/1 -> RT/1
  Oscillator/1(Out1) -> Complex to Real-Imag1/1
  Carrier Filter/1(Out1) -> filter error/1, Oscillator/1(phase error)
  Integrate and Dump4/1 -> "Carrier Loop  Discriminator "/2(Q_P), Display3/1
  Integrate and Dump1/1 -> Display/1, Data/1, "Carrier Loop  Discriminator "/1(I_P), Display2/1
  "PRN Generator "/4(code_phase_error) -> ?
  "PRN Generator "/5(code_phase_counter) -> code_phase_error/1
  Code Loop  Discriminator/1(error) -> "PRN Generator "/2(error)

== system Tracking/Tracking Loop/Tracking Loops/Tracking Loop1/Carrier Filter ==
  In2 : Inport
  Add : Sum
  Constant1 : Constant  Value=-1
  Constant2 : Constant
  Constant3 : Constant  Value=-1
  Delay : Delay  DelayLength=1  InitialCondition=0  SampleTime=0.001
  Discrete FIR Filter : DiscreteFir  CoefSource=Input port  Coefficients=[2 1]  SampleTime=0.001
      settings: InputPortMap=u0,u1
  Discrete Filter : DiscreteFilter  NumeratorSource=Input port  DenominatorSource=Input port  SampleTime=0.001  a0EqualsOne=on
      settings: InputPortMap=u0,p1,p3
  Product2 : Product
  Product3 : Product
  Product4 : Product
  Subsystem : Subsystem
  Sum : Sum  Inputs=|++
  Sum1 : Sum  Inputs=|++
  Vector Concatenate : Concatenate
  Vector Concatenate1 : Concatenate
  Out1 : Outport
  wires:
  Product2/1 -> Sum/1
  Sum/1 -> Delay/1, Sum1/1
  Delay/1 -> Sum/2
  Product3/1 -> Sum1/2
  Subsystem/1("K2 ") -> Add/1, Product2/2
  Subsystem/2(K1) -> Product4/1, Add/2, Product3/1
  In2/1 -> Discrete Filter/1, Discrete FIR Filter/1, Product3/2, Product2/1
  Vector Concatenate/1 -> Discrete Filter/2, Discrete FIR Filter/2
  Constant1/1 -> Product4/2
  Product4/1 -> Vector Concatenate/2
  Add/1 -> Vector Concatenate/1
  Discrete Filter/1 -> Out1/1
  Constant2/1 -> Vector Concatenate1/1
  Constant3/1 -> Vector Concatenate1/2
  Vector Concatenate1/1 -> Discrete Filter/3

== system Tracking/Tracking Loop/Tracking Loops/Tracking Loop1/Carrier Loop  Discriminator  ==
  I_P : Inport
  Q_P : Inport  Port=2
  Constant : Constant  Value=2*pi
  Divide : Product  Inputs=/*
  Divide1 : Product  Inputs=*/
  IC : InitialCondition  Value=0
  IC1 : InitialCondition
  IC2 : InitialCondition
  atan : Trigonometry  Operator=atan
  theta : Outport
  wires:
  atan/1 -> Divide1/1
  Divide/1 -> atan/1
  I_P/1 -> IC1/1
  IC/1 -> theta/1
  Constant/1 -> Divide1/2
  Divide1/1 -> IC/1
  Q_P/1 -> IC2/1
  IC1/1 -> Divide/1
  IC2/1 -> Divide/2

== system Tracking/Tracking Loop/Tracking Loops/Tracking Loop1/Code Loop  Discriminator ==
  I_E : Inport
  I_L : Inport  Port=2
  Q_E : Inport  Port=3
  Q_L : Inport  Port=4
  Add : Sum
  Add1 : Sum
  Add2 : Sum  Inputs=+-
  Add3 : Sum
  Display : Display
  Divide : Product  Inputs=*/
  IC : InitialCondition  Value=0
  Math Function{,2..3,5} (4 alike) : Math  Operator=magnitude^2  RndMeth=Zero  SaturateOnIntegerOverflow=on
  Sqrt : Sqrt  SaturateOnIntegerOverflow=on
  Sqrt1 : Sqrt  SaturateOnIntegerOverflow=on
  error : Outport  SampleTime=0.001
  wires:
  I_L/1 -> Math Function2/1
  I_E/1 -> Math Function/1
  Q_E/1 -> Math Function3/1
  Q_L/1 -> Math Function5/1
  Math Function2/1 -> Add1/1
  Math Function5/1 -> Add1/2
  Math Function/1 -> Add/1
  Math Function3/1 -> Add/2
  Add2/1 -> Divide/1
  Divide/1 -> IC/1
  IC/1 -> Display/1, error/1
  Add/1 -> Sqrt/1
  Add1/1 -> Sqrt1/1
  Sqrt/1 -> Add3/1, Add2/1
  Sqrt1/1 -> Add3/2, Add2/2
  Add3/1 -> Divide/2

== system Tracking/Tracking Loop/Tracking Loops/Tracking Loop1/Oscillator ==
  phase error : Inport
  Acq Freq : Inport  Port=2
  2*pi2 : Constant  Value=2*pi
  2^N2 : Constant  Value=2^16
  Add : Sum
  Counter Free-Running : simulink/Sources/Counter Free-Running  NumBits=15  tsamp=1/32768000
  Divide1 : Product  Inputs=*/
  Divide10 : Product
  Divide8 : Product  Inputs=*/*
  Divide9 : Product  Inputs=***
  Fs2 : Constant  Value=32768000
  IC : InitialCondition  Value=9207000
  MATLAB Function2 : MATLAB Function  TreatAsAtomicUnit=on
  Math Function : Math  Operator=mod  SaturateOnIntegerOverflow=on
  Pulse Generator1 : DiscretePulseGenerator  PulseType=Time based  Period=0.005  PulseWidth=50
  RT2 : RateTransition
  Real-Imag to Complex2 : RealImagToComplex
  Resettable Delay : Delay  DelayLength=1  ExternalReset=Rising  SampleTime=0.001
      settings: InputPortMap=u0,r5
  Sum2 : Sum  Inputs=-+|
  Out1 : Outport
  wires:
  2*pi2/1 -> Divide9/3, Divide10/1
  Sum2/1 -> Divide9/1
  Divide8/1 -> Sum2/2
  2^N2/1 -> Divide10/2, Divide1/2, Divide9/2
  Fs2/1 -> Divide8/2
  Divide10/1 -> Math Function/2
  phase error/1 -> Sum2/1
  Acq Freq/1 -> Divide8/1
  Pulse Generator1/1 -> RT2/1
  MATLAB Function2/1(I) -> Real-Imag to Complex2/1
  MATLAB Function2/2(Q) -> Real-Imag to Complex2/2
  Divide1/1 -> IC/1
  IC/1 -> MATLAB Function2/1(u)
  Resettable Delay/1 -> Add/1
  Math Function/1 -> Resettable Delay/1, Divide1/1
  Add/1 -> Math Function/1
  Divide9/1 -> Add/2
  Real-Imag to Complex2/1 -> Out1/1
  Counter Free-Running/1 -> Divide8/3

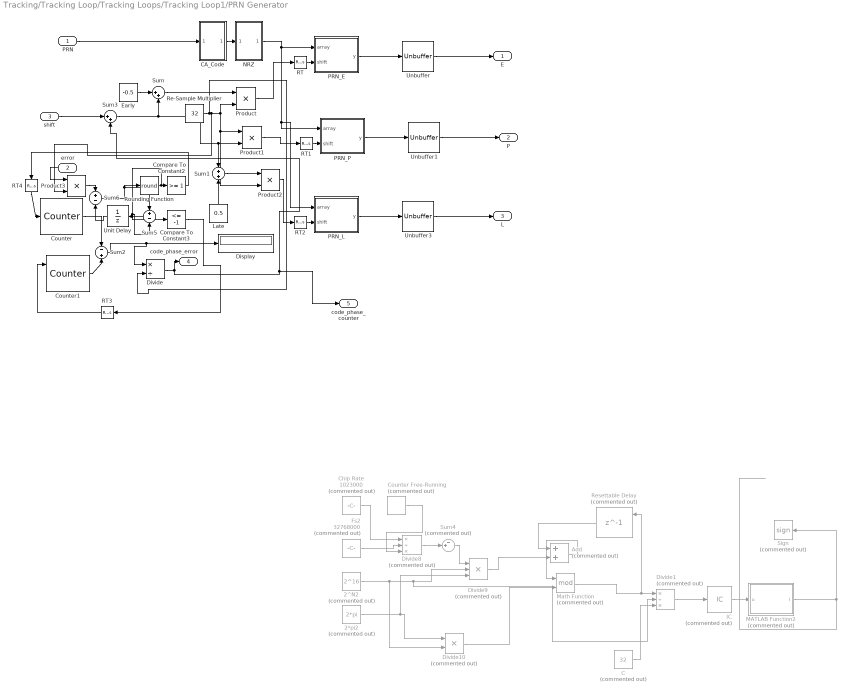
== system Tracking/Tracking Loop/Tracking Loops/Tracking Loop1/PRN Generator  ==
  PRN : Inport
  error : Inport  Port=2  SampleTime=0.001
  shift : Inport  Port=3
  2*pi2 : Constant  Commented=on  Value=2*pi
  2^N2 : Constant  Commented=on  Value=2^16
  Add : Sum  Commented=on
  C : Constant  Commented=on  Value=32
  "CA_Code " : Subsystem
  Chip Rate : Constant  Commented=on  Value=1023000
  Compare To Constant2 : simulink/Logic and Bit Operations/Compare To Constant  relop=>=  const=1  OutDataTypeStr=uint8
  Compare To Constant3 : simulink/Logic and Bit Operations/Compare To Constant  relop=<=  const=-1  OutDataTypeStr=uint8
  Counter : dspswit3/Counter  Direction=Up  CountEvent=Non-zero sample  CounterSize=User defined  MaxCount=2^16  InitialCount=0  Output=Count  HitValue=32  ResetInput=off  SamplesPerFrame=1  Ts=1  CntDtype=double  HitDtype=Logical
  Counter Free-Running : simulink/Sources/Counter Free-Running  Commented=on  NumBits=15  tsamp=1/32768000
  Counter1 : dspswit3/Counter  Direction=Up  CountEvent=Non-zero sample  CounterSize=User defined  MaxCount=2^16  InitialCount=0  Output=Count  HitValue=32  ResetInput=on  SamplesPerFrame=1  Ts=1  CntDtype=double  HitDtype=Logical
  Display : Display
  Divide : Product  Inputs=*/
  Divide1 : Product  Commented=on  Inputs=*/*
  Divide10 : Product  Commented=on
  Divide8 : Product  Commented=on  Inputs=*/*
  Divide9 : Product  Commented=on  Inputs=***
  Early : Constant  Value=-0.5
  Fs2 : Constant  Commented=on  Value=32768000
  IC : InitialCondition  Commented=on  Value=1023000
  Late : Constant  Value=0.5
  MATLAB Function2 : MATLAB Function  Commented=on  TreatAsAtomicUnit=on
  Math Function : Math  Commented=on  Operator=mod  SaturateOnIntegerOverflow=on
  NRZ : Subsystem
  PRN_E : MATLAB Function  TreatAsAtomicUnit=on  SystemSampleTime=0.001
  PRN_L : MATLAB Function  TreatAsAtomicUnit=on  SystemSampleTime=0.001
  PRN_P : MATLAB Function  TreatAsAtomicUnit=on  SystemSampleTime=0.001
  Product{,1..3} (4 alike) : Product
  RT{,1..4} (5 alike) : RateTransition  OutPortSampleTime=0.001
  Re-Sample Multiplier : Constant  Value=32
  Resettable Delay : Delay  Commented=on  DelayLength=1  ExternalReset=Rising  SampleTime=0.001
      settings: InputPortMap=u0,r5
  Rounding Function : Rounding  Operator=round
  Sign : Signum  Commented=on
  Sum : Sum  Inputs=|++
  Sum1 : Sum
  Sum2 : Sum  Inputs=-+
  Sum3 : Sum  Inputs=|++
  Sum4 : Sum  Commented=on  Inputs=-+|
  Sum5 : Sum  Inputs=+-
  Sum6 : Sum  Inputs=+-
  Unbuffer : Unbuffer
  Unbuffer1 : Unbuffer
  Unbuffer3 : Unbuffer
  Unit Delay : UnitDelay  SampleTime=0.001
  E : Outport
  P : Outport  Port=2
  L : Outport  Port=3
  code_phase_error : Outport  Port=4
  code_phase_counter : Outport  Port=5
  wires:
  Product/1 -> RT/1
  PRN_E/1(y) -> Unbuffer/1
  Product2/1 -> RT2/1
  PRN_L/1(y) -> Unbuffer3/1
  Re-Sample Multiplier/1 -> Divide/2, Product3/2, Product1/1, Product2/2, Product/2
  PRN/1 -> "CA_Code "/1(In1)
  Unbuffer1/1 -> P/1
  Unbuffer3/1 -> L/1
  Early/1 -> Sum/1
  Sum/1 -> Product/1
  Sum3/1 -> Product1/2, Sum1/1, Sum/2
  Sum1/1 -> Product2/1
  PRN_P/1(y) -> Unbuffer1/1
  error/1 -> Product3/1
  Counter/1 -> Sum2/1
  Counter1/1 -> Sum2/2
  Sum2/1 -> Divide/1, Display/1
  RT/1 -> PRN_E/2(shift)
  RT1/1 -> PRN_P/2(shift)
  RT2/1 -> PRN_L/2(shift)
  Late/1 -> Sum1/2
  "CA_Code "/1(Out1) -> NRZ/1(In1)
  Unbuffer/1 -> E/1
  NRZ/1(Out1) -> PRN_E/1(array), PRN_L/1(array), PRN_P/1(array)
  Product1/1 -> RT1/1
  MATLAB Function2/1(I) -> Sign/1
  Divide8/1 -> Sum4/2
  C/1 -> Divide1/3
  2^N2/1 -> Divide10/2, Divide1/2, Divide9/2
  Fs2/1 -> Divide8/2
  2*pi2/1 -> Divide9/3, Divide10/1
  Sum4/1 -> Divide9/1
  IC/1 -> MATLAB Function2/1(u)
  Divide10/1 -> Math Function/2
  Chip Rate/1 -> Divide8/1
  Resettable Delay/1 -> Add/1
  Divide1/1 -> IC/1
  Divide9/1 -> Add/2
  Counter Free-Running/1 -> Divide8/3
  Add/1 -> Math Function/1
  Math Function/1 -> Resettable Delay/1, Divide1/1
  Compare To Constant2/1 -> RT4/1
  Compare To Constant3/1 -> RT3/1
  Rounding Function/1 -> Sum5/2, Compare To Constant3/1, Compare To Constant2/1
  Product3/1 -> Sum6/1
  Sum5/1 -> Unit Delay/1
  Sum6/1 -> Sum5/1, Rounding Function/1
  Unit Delay/1 -> Sum6/2
  shift/1 -> Sum3/1
  Divide/1 -> Sum3/2, code_phase_counter/1, code_phase_error/1
  RT3/1 -> Counter1/1
  RT4/1 -> Counter/1

== system Tracking/Tracking Loop/Tracking Loops/Tracking Loop2/Carrier Filter ==
  In2 : Inport
  Add : Sum
  Constant1 : Constant  Value=-1
  Constant2 : Constant
  Constant3 : Constant  Value=-1
  Delay : Delay  DelayLength=1  InitialCondition=0  SampleTime=0.001
  Discrete FIR Filter : DiscreteFir  CoefSource=Input port  Coefficients=[2 1]  SampleTime=0.001
      settings: InputPortMap=u0,u1
  Discrete Filter : DiscreteFilter  NumeratorSource=Input port  DenominatorSource=Input port  SampleTime=0.001  a0EqualsOne=on
      settings: InputPortMap=u0,p1,p3
  Product2 : Product
  Product3 : Product
  Product4 : Product
  Subsystem : Subsystem
  Sum : Sum  Inputs=|++
  Sum1 : Sum  Inputs=|++
  Vector Concatenate : Concatenate
  Vector Concatenate1 : Concatenate
  Out1 : Outport
  wires:
  Product2/1 -> Sum/1
  Sum/1 -> Delay/1, Sum1/1
  Delay/1 -> Sum/2
  Product3/1 -> Sum1/2
  Subsystem/1("K2 ") -> Add/1, Product2/2
  Subsystem/2(K1) -> Product4/1, Add/2, Product3/1
  In2/1 -> Discrete Filter/1, Discrete FIR Filter/1, Product3/2, Product2/1
  Vector Concatenate/1 -> Discrete Filter/2, Discrete FIR Filter/2
  Constant1/1 -> Product4/2
  Product4/1 -> Vector Concatenate/2
  Add/1 -> Vector Concatenate/1
  Discrete Filter/1 -> Out1/1
  Constant2/1 -> Vector Concatenate1/1
  Constant3/1 -> Vector Concatenate1/2
  Vector Concatenate1/1 -> Discrete Filter/3

== system Tracking/Tracking Loop/Tracking Loops/Tracking Loop2/Carrier Loop  Discriminator  ==
  I_P : Inport
  Q_P : Inport  Port=2
  Constant : Constant  Value=2*pi
  Divide : Product  Inputs=/*
  Divide1 : Product  Inputs=*/
  IC : InitialCondition  Value=0
  IC1 : InitialCondition
  IC2 : InitialCondition
  atan : Trigonometry  Operator=atan
  theta : Outport
  wires:
  atan/1 -> Divide1/1
  Divide/1 -> atan/1
  I_P/1 -> IC1/1
  IC/1 -> theta/1
  Constant/1 -> Divide1/2
  Divide1/1 -> IC/1
  Q_P/1 -> IC2/1
  IC1/1 -> Divide/1
  IC2/1 -> Divide/2

== system Tracking/Tracking Loop/Tracking Loops/Tracking Loop2/Code Loop  Discriminator ==
  I_E : Inport
  I_L : Inport  Port=2
  Q_E : Inport  Port=3
  Q_L : Inport  Port=4
  Add : Sum
  Add1 : Sum
  Add2 : Sum  Inputs=+-
  Add3 : Sum
  Display : Display
  Divide : Product  Inputs=*/
  IC : InitialCondition  Value=0
  Math Function{,2..3,5} (4 alike) : Math  Operator=magnitude^2  RndMeth=Zero  SaturateOnIntegerOverflow=on
  Sqrt : Sqrt  SaturateOnIntegerOverflow=on
  Sqrt1 : Sqrt  SaturateOnIntegerOverflow=on
  error : Outport  SampleTime=0.001
  wires:
  I_L/1 -> Math Function2/1
  I_E/1 -> Math Function/1
  Q_E/1 -> Math Function3/1
  Q_L/1 -> Math Function5/1
  Math Function2/1 -> Add1/1
  Math Function5/1 -> Add1/2
  Math Function/1 -> Add/1
  Math Function3/1 -> Add/2
  Add2/1 -> Divide/1
  Divide/1 -> IC/1
  IC/1 -> Display/1, error/1
  Add/1 -> Sqrt/1
  Add1/1 -> Sqrt1/1
  Sqrt/1 -> Add3/1, Add2/1
  Sqrt1/1 -> Add3/2, Add2/2
  Add3/1 -> Divide/2

== system Tracking/Tracking Loop/Tracking Loops/Tracking Loop2/Oscillator ==
  phase error : Inport
  Acq Freq : Inport  Port=2
  2*pi2 : Constant  Value=2*pi
  2^N2 : Constant  Value=2^16
  Add : Sum
  Counter Free-Running : simulink/Sources/Counter Free-Running  NumBits=15  tsamp=1/32768000
  Divide1 : Product  Inputs=*/
  Divide10 : Product
  Divide8 : Product  Inputs=*/*
  Divide9 : Product  Inputs=***
  Fs2 : Constant  Value=32768000
  IC : InitialCondition  Value=9207000
  MATLAB Function2 : MATLAB Function  TreatAsAtomicUnit=on
  Math Function : Math  Operator=mod  SaturateOnIntegerOverflow=on
  Pulse Generator1 : DiscretePulseGenerator  PulseType=Time based  Period=0.005  PulseWidth=50
  RT2 : RateTransition
  Real-Imag to Complex2 : RealImagToComplex
  Resettable Delay : Delay  DelayLength=1  ExternalReset=Rising  SampleTime=0.001
      settings: InputPortMap=u0,r5
  Sum2 : Sum  Inputs=-+|
  Out1 : Outport
  wires:
  2*pi2/1 -> Divide9/3, Divide10/1
  Sum2/1 -> Divide9/1
  Divide8/1 -> Sum2/2
  2^N2/1 -> Divide10/2, Divide1/2, Divide9/2
  Fs2/1 -> Divide8/2
  Divide10/1 -> Math Function/2
  phase error/1 -> Sum2/1
  Acq Freq/1 -> Divide8/1
  Pulse Generator1/1 -> RT2/1
  MATLAB Function2/1(I) -> Real-Imag to Complex2/1
  MATLAB Function2/2(Q) -> Real-Imag to Complex2/2
  Divide1/1 -> IC/1
  IC/1 -> MATLAB Function2/1(u)
  Resettable Delay/1 -> Add/1
  Math Function/1 -> Resettable Delay/1, Divide1/1
  Add/1 -> Math Function/1
  Divide9/1 -> Add/2
  Real-Imag to Complex2/1 -> Out1/1
  Counter Free-Running/1 -> Divide8/3

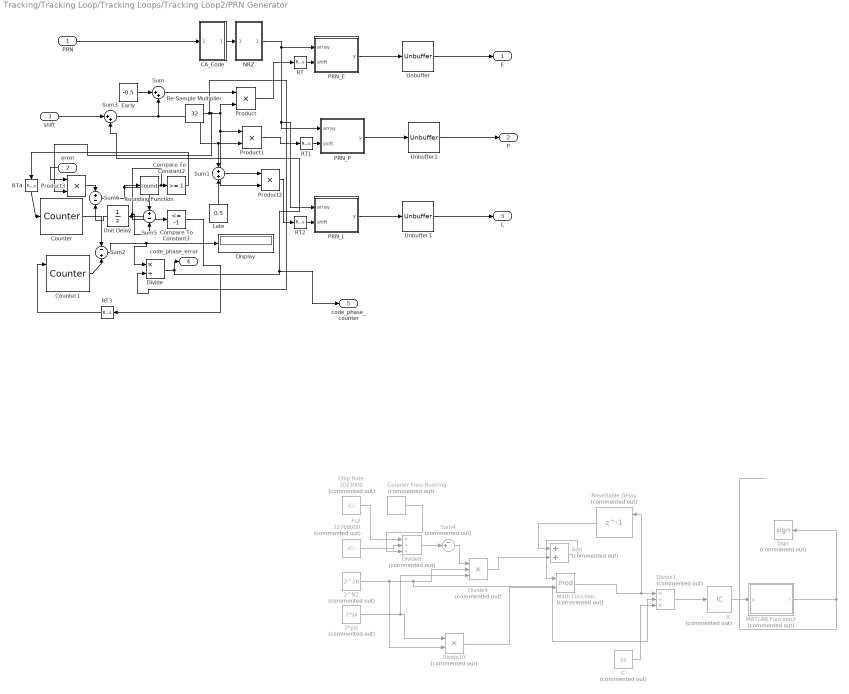
== system Tracking/Tracking Loop/Tracking Loops/Tracking Loop2/PRN Generator  ==
  PRN : Inport
  error : Inport  Port=2  SampleTime=0.001
  shift : Inport  Port=3
  2*pi2 : Constant  Commented=on  Value=2*pi
  2^N2 : Constant  Commented=on  Value=2^16
  Add : Sum  Commented=on
  C : Constant  Commented=on  Value=32
  "CA_Code " : Subsystem
  Chip Rate : Constant  Commented=on  Value=1023000
  Compare To Constant2 : simulink/Logic and Bit Operations/Compare To Constant  relop=>=  const=1  OutDataTypeStr=uint8
  Compare To Constant3 : simulink/Logic and Bit Operations/Compare To Constant  relop=<=  const=-1  OutDataTypeStr=uint8
  Counter : dspswit3/Counter  Direction=Up  CountEvent=Non-zero sample  CounterSize=User defined  MaxCount=2^16  InitialCount=0  Output=Count  HitValue=32  ResetInput=off  SamplesPerFrame=1  Ts=1  CntDtype=double  HitDtype=Logical
  Counter Free-Running : simulink/Sources/Counter Free-Running  Commented=on  NumBits=15  tsamp=1/32768000
  Counter1 : dspswit3/Counter  Direction=Up  CountEvent=Non-zero sample  CounterSize=User defined  MaxCount=2^16  InitialCount=0  Output=Count  HitValue=32  ResetInput=on  SamplesPerFrame=1  Ts=1  CntDtype=double  HitDtype=Logical
  Display : Display
  Divide : Product  Inputs=*/
  Divide1 : Product  Commented=on  Inputs=*/*
  Divide10 : Product  Commented=on
  Divide8 : Product  Commented=on  Inputs=*/*
  Divide9 : Product  Commented=on  Inputs=***
  Early : Constant  Value=-0.5
  Fs2 : Constant  Commented=on  Value=32768000
  IC : InitialCondition  Commented=on  Value=1023000
  Late : Constant  Value=0.5
  MATLAB Function2 : MATLAB Function  Commented=on  TreatAsAtomicUnit=on
  Math Function : Math  Commented=on  Operator=mod  SaturateOnIntegerOverflow=on
  NRZ : Subsystem
  PRN_E : MATLAB Function  TreatAsAtomicUnit=on  SystemSampleTime=0.001
  PRN_L : MATLAB Function  TreatAsAtomicUnit=on  SystemSampleTime=0.001
  PRN_P : MATLAB Function  TreatAsAtomicUnit=on  SystemSampleTime=0.001
  Product{,1..3} (4 alike) : Product
  RT{,1..4} (5 alike) : RateTransition  OutPortSampleTime=0.001
  Re-Sample Multiplier : Constant  Value=32
  Resettable Delay : Delay  Commented=on  DelayLength=1  ExternalReset=Rising  SampleTime=0.001
      settings: InputPortMap=u0,r5
  Rounding Function : Rounding  Operator=round
  Sign : Signum  Commented=on
  Sum : Sum  Inputs=|++
  Sum1 : Sum
  Sum2 : Sum  Inputs=-+
  Sum3 : Sum  Inputs=|++
  Sum4 : Sum  Commented=on  Inputs=-+|
  Sum5 : Sum  Inputs=+-
  Sum6 : Sum  Inputs=+-
  Unbuffer : Unbuffer
  Unbuffer1 : Unbuffer
  Unbuffer3 : Unbuffer
  Unit Delay : UnitDelay  SampleTime=0.001
  E : Outport
  P : Outport  Port=2
  L : Outport  Port=3
  code_phase_error : Outport  Port=4
  code_phase_counter : Outport  Port=5
  wires:
  Product/1 -> RT/1
  PRN_E/1(y) -> Unbuffer/1
  Product2/1 -> RT2/1
  PRN_L/1(y) -> Unbuffer3/1
  Re-Sample Multiplier/1 -> Divide/2, Product3/2, Product1/1, Product2/2, Product/2
  PRN/1 -> "CA_Code "/1(In1)
  Unbuffer1/1 -> P/1
  Unbuffer3/1 -> L/1
  Early/1 -> Sum/1
  Sum/1 -> Product/1
  Sum3/1 -> Product1/2, Sum1/1, Sum/2
  Sum1/1 -> Product2/1
  PRN_P/1(y) -> Unbuffer1/1
  error/1 -> Product3/1
  Counter/1 -> Sum2/1
  Counter1/1 -> Sum2/2
  Sum2/1 -> Divide/1, Display/1
  RT/1 -> PRN_E/2(shift)
  RT1/1 -> PRN_P/2(shift)
  RT2/1 -> PRN_L/2(shift)
  Late/1 -> Sum1/2
  "CA_Code "/1(Out1) -> NRZ/1(In1)
  Unbuffer/1 -> E/1
  NRZ/1(Out1) -> PRN_E/1(array), PRN_L/1(array), PRN_P/1(array)
  Product1/1 -> RT1/1
  MATLAB Function2/1(I) -> Sign/1
  Divide8/1 -> Sum4/2
  C/1 -> Divide1/3
  2^N2/1 -> Divide10/2, Divide1/2, Divide9/2
  Fs2/1 -> Divide8/2
  2*pi2/1 -> Divide9/3, Divide10/1
  Sum4/1 -> Divide9/1
  IC/1 -> MATLAB Function2/1(u)
  Divide10/1 -> Math Function/2
  Chip Rate/1 -> Divide8/1
  Resettable Delay/1 -> Add/1
  Divide1/1 -> IC/1
  Divide9/1 -> Add/2
  Counter Free-Running/1 -> Divide8/3
  Add/1 -> Math Function/1
  Math Function/1 -> Resettable Delay/1, Divide1/1
  Compare To Constant2/1 -> RT4/1
  Compare To Constant3/1 -> RT3/1
  Rounding Function/1 -> Sum5/2, Compare To Constant3/1, Compare To Constant2/1
  Product3/1 -> Sum6/1
  Sum5/1 -> Unit Delay/1
  Sum6/1 -> Sum5/1, Rounding Function/1
  Unit Delay/1 -> Sum6/2
  shift/1 -> Sum3/1
  Divide/1 -> Sum3/2, code_phase_counter/1, code_phase_error/1
  RT3/1 -> Counter1/1
  RT4/1 -> Counter/1

== system Tracking/Tracking Loop/Tracking Loops/Tracking Loop3/Carrier Filter ==
  In2 : Inport
  Add : Sum
  Constant1 : Constant  Value=-1
  Constant2 : Constant
  Constant3 : Constant  Value=-1
  Delay : Delay  DelayLength=1  InitialCondition=0  SampleTime=0.001
  Discrete FIR Filter : DiscreteFir  CoefSource=Input port  Coefficients=[2 1]  SampleTime=0.001
      settings: InputPortMap=u0,u1
  Discrete Filter : DiscreteFilter  NumeratorSource=Input port  DenominatorSource=Input port  SampleTime=0.001  a0EqualsOne=on
      settings: InputPortMap=u0,p1,p3
  Product2 : Product
  Product3 : Product
  Product4 : Product
  Subsystem : Subsystem
  Sum : Sum  Inputs=|++
  Sum1 : Sum  Inputs=|++
  Vector Concatenate : Concatenate
  Vector Concatenate1 : Concatenate
  Out1 : Outport
  wires:
  Product2/1 -> Sum/1
  Sum/1 -> Delay/1, Sum1/1
  Delay/1 -> Sum/2
  Product3/1 -> Sum1/2
  Subsystem/1("K2 ") -> Add/1, Product2/2
  Subsystem/2(K1) -> Product4/1, Add/2, Product3/1
  In2/1 -> Discrete Filter/1, Discrete FIR Filter/1, Product3/2, Product2/1
  Vector Concatenate/1 -> Discrete Filter/2, Discrete FIR Filter/2
  Constant1/1 -> Product4/2
  Product4/1 -> Vector Concatenate/2
  Add/1 -> Vector Concatenate/1
  Discrete Filter/1 -> Out1/1
  Constant2/1 -> Vector Concatenate1/1
  Constant3/1 -> Vector Concatenate1/2
  Vector Concatenate1/1 -> Discrete Filter/3

== system Tracking/Tracking Loop/Tracking Loops/Tracking Loop3/Carrier Loop  Discriminator  ==
  I_P : Inport
  Q_P : Inport  Port=2
  Constant : Constant  Value=2*pi
  Divide : Product  Inputs=/*
  Divide1 : Product  Inputs=*/
  IC : InitialCondition  Value=0
  IC1 : InitialCondition
  IC2 : InitialCondition
  atan : Trigonometry  Operator=atan
  theta : Outport
  wires:
  atan/1 -> Divide1/1
  Divide/1 -> atan/1
  I_P/1 -> IC1/1
  IC/1 -> theta/1
  Constant/1 -> Divide1/2
  Divide1/1 -> IC/1
  Q_P/1 -> IC2/1
  IC1/1 -> Divide/1
  IC2/1 -> Divide/2

== system Tracking/Tracking Loop/Tracking Loops/Tracking Loop3/Code Loop  Discriminator ==
  I_E : Inport
  I_L : Inport  Port=2
  Q_E : Inport  Port=3
  Q_L : Inport  Port=4
  Add : Sum
  Add1 : Sum
  Add2 : Sum  Inputs=+-
  Add3 : Sum
  Display : Display
  Divide : Product  Inputs=*/
  IC : InitialCondition  Value=0
  Math Function{,2..3,5} (4 alike) : Math  Operator=magnitude^2  RndMeth=Zero  SaturateOnIntegerOverflow=on
  Sqrt : Sqrt  SaturateOnIntegerOverflow=on
  Sqrt1 : Sqrt  SaturateOnIntegerOverflow=on
  error : Outport  SampleTime=0.001
  wires:
  I_L/1 -> Math Function2/1
  I_E/1 -> Math Function/1
  Q_E/1 -> Math Function3/1
  Q_L/1 -> Math Function5/1
  Math Function2/1 -> Add1/1
  Math Function5/1 -> Add1/2
  Math Function/1 -> Add/1
  Math Function3/1 -> Add/2
  Add2/1 -> Divide/1
  Divide/1 -> IC/1
  IC/1 -> Display/1, error/1
  Add/1 -> Sqrt/1
  Add1/1 -> Sqrt1/1
  Sqrt/1 -> Add3/1, Add2/1
  Sqrt1/1 -> Add3/2, Add2/2
  Add3/1 -> Divide/2
